simulink model "InvertedPendulum"  (R2024b)
settings: Solver=VariableStepAuto  StartTime=0.0  StopTime=inf  FixedStep=0.001  RelTol=1e-3
model workspace (MAT data in the model file):
  Sig = Simulink.Signal
  Sig.Dimensions = -1
  Sig.DimensionsMode = 'auto'
  Sig.Complexity = 'auto'
  Sig.SampleTime = -1
  Sig.SamplingMode = 'auto'
  Sig.DataType = 'auto'
libraries: simulink x4
settings Model: Creator=nopla  LastModifiedBy=nop
settings OptimizationCC: DefaultParameterBehavior=Inlined  UseDivisionForNetSlopeComputation=on  GainParamInheritBuiltInType=on  UseFloatMulNetSlope=on  EnhancedBackFolding=on  PassReuseOutputArgsAs=Individual arguments  ZeroExternalMemoryAtStartup=off  ZeroInternalMemoryAtStartup=off  EfficientFloat2IntCast=on  OptimizeBlockOrder=speed  DifferentSizesBufferReuse=on  EfficientTunableParamExpr=on
settings DebuggingCC: ParameterTunabilityLossMsg=error
settings HardwareCC: ProdLongLongMode=on
settings SFSimCC: MATLABDynamicMemAlloc=off
settings RTWCC: Description=Embedded Coder  SystemTargetFile=ert.tlc  GenCodeOnly=on  TemplateMakefile=ert_default_tmf  GenerateReport=on  LaunchReport=on
settings CodeAppCC: ForceParamTrailComments=on  IgnoreCustomStorageClasses=off  OperatorAnnotations=on  SimulinkDataObjDesc=on  SFDataObjDesc=on  InsertBlockDesc=on
settings ERTTargetCC: TargetLangStandard=C99 (ISO)  GenerateSampleERTMain=on  ERTCustomFileTemplate=example_file_process.tlc

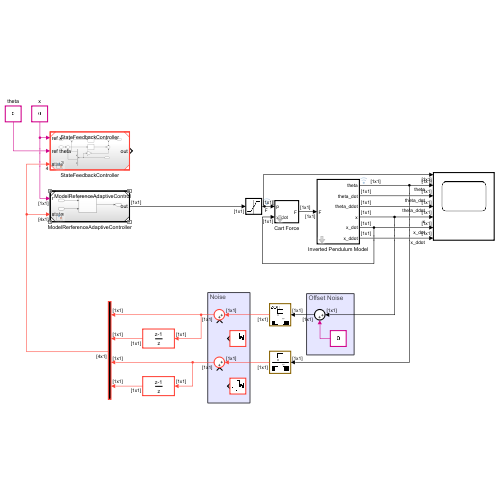
[thumbnail: Simulink's stored preview of the top-level diagram]
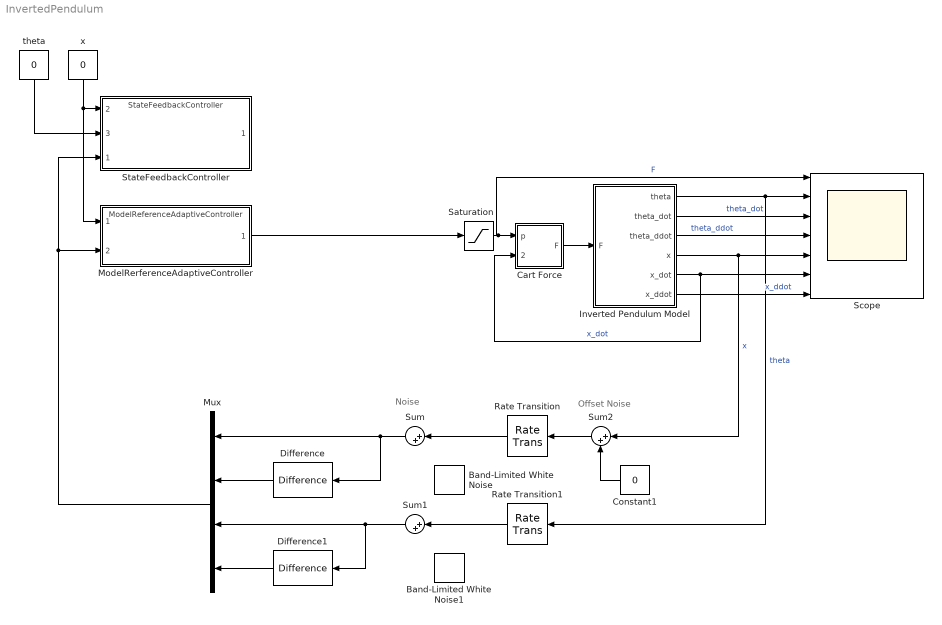
== system InvertedPendulum ==
  note: Noise
  note: Offset Noise
  Band-Limited White Noise : simulink/Sources/Band-Limited White Noise  Cov=[0.002]  Ts=0.001  seed=[23341]
  Band-Limited White Noise1 : simulink/Sources/Band-Limited White Noise  Cov=[0.0001]  Ts=0.001  seed=[23341]
  Cart Force : Subsystem  mask{omega_max=523.6*0.6, tau_max=0.030*0.6, G=6.67, r=0.0255}
      mask prompts: omega_max "モータ最大回転数"; tau_max "モータ最大トルク"; G "減速比"; r "タイヤ半径"
      mask DialogControl ParameterGroupVar Prompt: パラメーター
  Constant1 : Constant  Value=0
  Difference : simulink/Discrete/Difference  ICPrevInput=0.0  OutMin=[]  OutMax=[]  OutDataType=fixdt(1, 16)  OutScaling=2^-10  DoSatur=off
  Difference1 : simulink/Discrete/Difference  ICPrevInput=0.0  OutMin=[]  OutMax=[]  OutDataType=fixdt(1, 16)  OutScaling=2^-10  DoSatur=off
  Inverted Pendulum Model : Subsystem  mask{CartMass=0.698, PendulumMass=0.0303, PendulumLength=0.15, PendulumInertia=(1/3)*0.0303*0.15^2, g=9.81, ThetaInitialValue=0, XInitialValue=0}
      mask prompts: ThetaInitialValue "初期値 x"; XInitialValue "初期値 theta"
      mask DialogControl ParameterGroupVar Prompt: パラメーター
  ModelRerferenceAdaptiveController : ModelReference  ModelNameDialog=ModelReferenceAdaptiveController.slx  SimulationMode=Normal  ModelReferenceVersion=1.5
  Mux : Mux
  Rate Transition : RateTransition  OutPortSampleTime=0.001
  Rate Transition1 : RateTransition  OutPortSampleTime=0.001
  Saturation : Saturate  UpperLimit=1  LowerLimit=-1
  Scope : Scope  NumInputPorts=7
  StateFeedbackController : ModelReference  ModelNameDialog=StateFeedbackController.slx  SimulationMode=Normal  ModelReferenceVersion=1.223
      settings: PortSchema="{\"entries\":[{\"content\":{\"sides\":[{\"content\":{\"connectorIds\":[\"In2\",\"In3\",\"In1\"]},\"type\":\"ConnectorPlacement.EquallySpacedRectSide\",\"uuid\":\"6e4d8e87-2093-4045-b6f4-9c4eed5b36da\"},{\"content\":{\"connectorIds\":[\"Out1\"],\"side\":\"RIGHT\"},\"type\":\"ConnectorPlacement.EquallySpacedRectSide\",\"uuid\":\"38b84323-b42e-4c2d-81dd-b76627ceba1d\"},{\"content\":{\"side\":\"TOP\"},\"type\":\"ConnectorPlacement.EquallySpacedRectSide\",\"uuid\":\"25faced0-4653-476f-8031-70bb4df7532c\"}]},\"type\":\"ConnectorPlacement.EquallySpacedConnector\",\"uuid\":\"92f29b28-6892-435d-8b82-1b99566fda4e\"}],\"packageUris\":[\"http://schema.mathworks.com/mf0/Connector/R2020b\"],\"version\":\"1.0\"}"
  Sum : Sum  Inputs=|++
  Sum1 : Sum  Inputs=|++
  Sum2 : Sum  Inputs=|++
  theta : Constant  Value=0
  x : Constant  Value=0
  wires:
  Inverted Pendulum Model/1(theta) -> Rate Transition1/1, Scope/2  "theta"
  Inverted Pendulum Model/2(theta_dot) -> Scope/3  "theta_dot"
  Inverted Pendulum Model/3(theta_ddot) -> Scope/4  "theta_ddot"
  Inverted Pendulum Model/4(x) -> Sum2/1, Scope/5  "x"
  Inverted Pendulum Model/5(x_dot) -> Cart Force/2(x_dot), Scope/6  "x_dot"
  Inverted Pendulum Model/6(x_ddot) -> Scope/7  "x_ddot"
  Cart Force/1(F) -> Inverted Pendulum Model/1(F)
  Difference/1 -> Mux/2
  Difference1/1 -> Mux/4
  Rate Transition/1 -> Sum/1
  Sum/1 -> Mux/1, Difference/1
  Rate Transition1/1 -> Sum1/1
  Sum1/1 -> Mux/3, Difference1/1
  Sum2/1 -> Rate Transition/1
  Constant1/1 -> Sum2/2
  Mux/1 -> ModelRerferenceAdaptiveController/2, StateFeedbackController/1
  x/1 -> StateFeedbackController/2, ModelRerferenceAdaptiveController/1
  Saturation/1 -> Scope/1, Cart Force/1(p)  "F"
  theta/1 -> StateFeedbackController/3
  ModelRerferenceAdaptiveController/1 -> Saturation/1

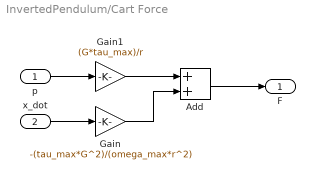
== system InvertedPendulum/Cart Force ==
  p : Inport
  x_dot : Inport  Port=2
  Add : Sum
  Gain : Gain  Gain=-(tau_max*G^2)/(omega_max*r^2)
  Gain1 : Gain  Gain=(G*tau_max)/r
  F : Outport
  wires:
  x_dot/1 -> Gain/1
  Gain1/1 -> Add/1
  Gain/1 -> Add/2
  Add/1 -> F/1
  p/1 -> Gain1/1

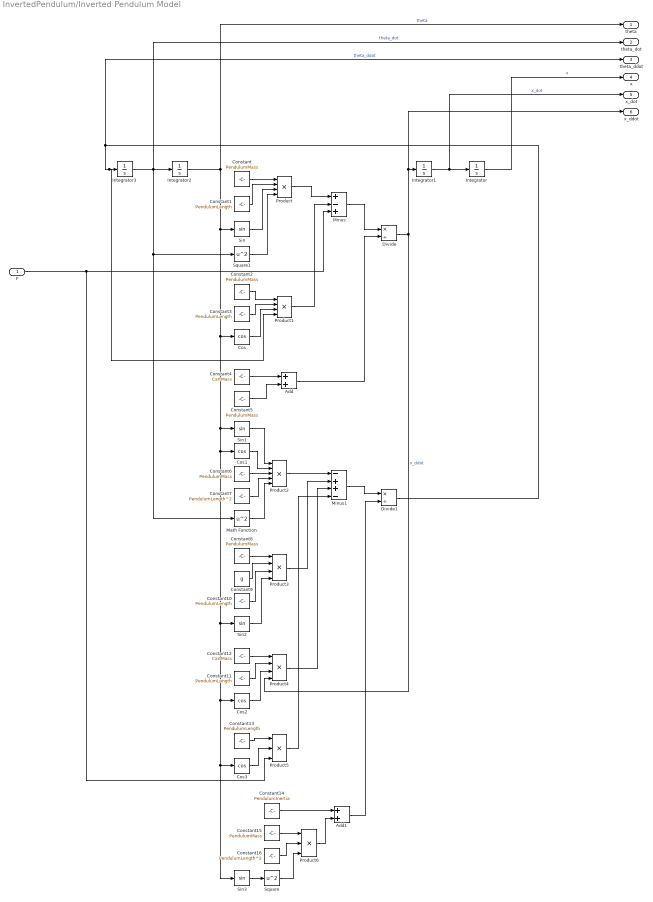
== system InvertedPendulum/Inverted Pendulum Model ==
  F : Inport
  Add : Sum
  Add1 : Sum
  Constant{,2,5..6,8,15} (6 alike) : Constant  Value=PendulumMass
  Constant{1,3,10..11,13} (5 alike) : Constant  Value=PendulumLength
  Constant12 : Constant  Value=CartMass
  Constant14 : Constant  Value=PendulumInertia
  Constant16 : Constant  Value=PendulumLength^2
  Constant4 : Constant  Value=CartMass
  Constant7 : Constant  Value=PendulumLength^2
  Constant9 : Constant  Value=g
  Cos{,1..3} (4 alike) : Trigonometry  Operator=cos
  Divide : Product  Inputs=*/
  Divide1 : Product  Inputs=*/
  Integrator : Integrator  InitialCondition=XInitialValue
  Integrator1 : Integrator
  Integrator2 : Integrator  InitialCondition=ThetaInitialValue
  Integrator3 : Integrator
  Math Function : Math  Operator=square
  Minus : Sum  Inputs=+-+
  Minus1 : Sum  Inputs=-++-
  Product{,1,3..4} (4 alike) : Product  Inputs=4
  Product2 : Product  Inputs=5
  Product5 : Product  Inputs=3
  Product6 : Product  Inputs=3
  Sin{,1..3} (4 alike) : Trigonometry
  Square : Math  Operator=square
  Square1 : Math  Operator=square
  theta : Outport
  theta_dot : Outport  Port=2
  theta_ddot : Outport  Port=3
  x : Outport  Port=4
  x_dot : Outport  Port=5
  x_ddot : Outport  Port=6
  wires:
  Square/1 -> Product6/3
  Integrator2/1 -> theta/1, Cos2/1, Sin3/1, Cos3/1, Sin2/1, Cos1/1, Sin1/1, Cos/1, Sin/1  "theta"
  Product6/1 -> Add1/2
  Sin2/1 -> Product3/4
  Minus1/1 -> Divide1/1
  Integrator3/1 -> theta_dot/1, Math Function/1, Square1/1, Integrator2/1  "theta_dot"
  Constant15/1 -> Product6/1
  Cos/1 -> Product1/3
  Constant10/1 -> Product3/3
  Cos2/1 -> Product4/3
  Constant12/1 -> Product4/1
  Constant1/1 -> Product/2
  Divide/1 -> Product4/4, x_ddot/1, Integrator1/1  "x_ddot"
  F/1 -> Minus/3, Product5/3
  Integrator/1 -> x/1  "x"
  Constant3/1 -> Product1/2
  Integrator1/1 -> x_dot/1, Integrator/1  "x_dot"
  Sin3/1 -> Square/1
  Product2/1 -> Minus1/1
  Product5/1 -> Minus1/4
  Constant16/1 -> Product6/2
  Constant4/1 -> Add/1
  Product1/1 -> Minus/2
  Constant7/1 -> Product2/4
  Constant9/1 -> Product3/2
  Product3/1 -> Minus1/2
  Add1/1 -> Divide1/2
  Square1/1 -> Product/4
  Sin1/1 -> Product2/1
  Constant/1 -> Product/1
  Sin/1 -> Product/3
  Cos3/1 -> Product5/2
  Divide1/1 -> theta_ddot/1, Integrator3/1, Product1/4  "theta_ddot"
  Constant5/1 -> Add/2
  Constant14/1 -> Add1/1
  Add/1 -> Divide/2
  Constant2/1 -> Product1/1
  Math Function/1 -> Product2/5
  Product/1 -> Minus/1
  Constant8/1 -> Product3/1
  Minus/1 -> Divide/1
  Constant11/1 -> Product4/2
  Constant6/1 -> Product2/3
  Product4/1 -> Minus1/3
  Cos1/1 -> Product2/2
  Constant13/1 -> Product5/1
